simulink model "traditional"  (R2020b)
settings: Solver=FixedStepAuto  StartTime=0.0  StopTime=5  FixedStep=0.001  RelTol=1e-3
libraries: simulink x1
settings Model: Creator=up!  LastModifiedBy=up!

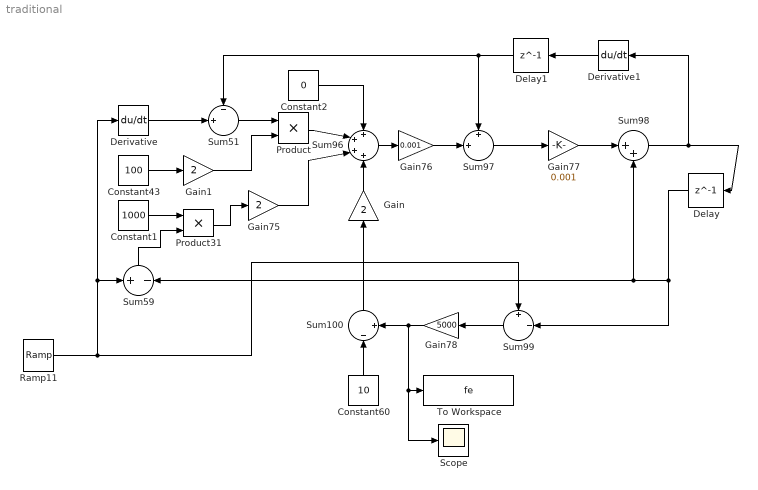
== system traditional ==
  Constant1 : Constant  Value=1000
  Constant2 : Constant  Value=0
  Constant43 : Constant  Value=100
  Constant60 : Constant  Value=10
  Delay : Delay  DelayLength=1  InitialCondition=0
  Delay1 : Delay  DelayLength=1  InitialCondition=0
  Derivative : Derivative
  Derivative1 : Derivative
  Gain : Gain  Gain=2
  Gain1 : Gain  Gain=2
  Gain75 : Gain  Gain=2
  Gain76 : Gain  Gain=0.001
  Gain77 : Gain  Gain=0.001
  Gain78 : Gain  Gain=5000
  Product : Product
  Product31 : Product
  Ramp11 : simulink/Sources/Ramp  slope=0.1  start=0  InitialOutput=0
  Scope : Scope
  Sum100 : Sum  Inputs=||-|+
  Sum51 : Sum  Inputs=-|+||
  Sum59 : Sum  Inputs=+-
  Sum96 : Sum  Inputs=++++
  Sum97 : Sum  Inputs=+|+||
  Sum98 : Sum  Inputs=|++
  Sum99 : Sum  Inputs=+|-||
  To Workspace : ToWorkspace  VariableName=fe  SaveFormat=Timeseries  SampleTime=-1
  wires:
  Sum96/1 -> Gain76/1
  Gain76/1 -> Sum97/2
  Ramp11/1 -> Sum59/1, Derivative/1, Sum99/1
  Product31/1 -> Gain75/1
  Gain/1 -> Sum96/4
  Derivative/1 -> Sum51/2
  Gain75/1 -> Sum96/3
  Sum97/1 -> Gain77/1
  Delay1/1 -> Sum51/1, Sum97/1
  Gain1/1 -> Product/2
  Sum100/1 -> Gain/1
  Sum99/1 -> Gain78/1
  Sum51/1 -> Product/1
  Product/1 -> Sum96/2
  Constant2/1 -> Sum96/1
  Sum98/1 -> Delay/1, Derivative1/1
  Delay/1 -> Sum99/2, Sum98/2, Sum59/2
  Sum59/1 -> Product31/2
  Derivative1/1 -> Delay1/1
  Gain77/1 -> Sum98/1
  Constant43/1 -> Gain1/1
  Constant1/1 -> Product31/1
  Constant60/1 -> Sum100/1
  Gain78/1 -> Scope/1, To Workspace/1, Sum100/2
